simulink model "complex_addsub_test"  (Simulink 7.0)
settings: Solver=VariableStepDiscrete  StartTime=0.0  StopTime=1000  RelTol=1e-3
libraries: xbsIndex_r4 x13, casper_library x5
settings Model: Creator=User  LastModifiedBy=User
settings DebuggingCC: SaveWithDisabledLinksMsg=none  SaveWithParameterizedLinksMsg=none

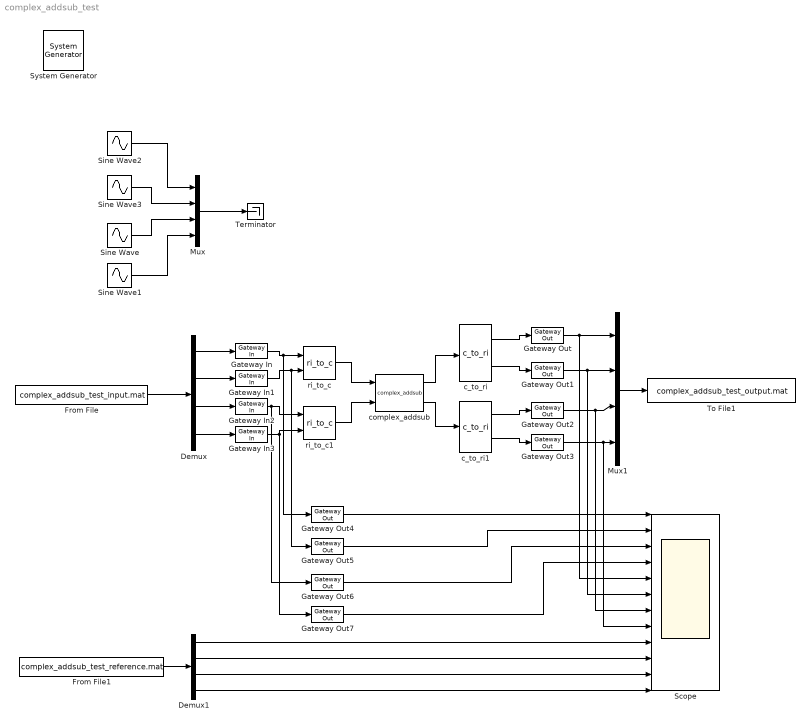
== system complex_addsub_test ==
  " System Generator" : xbsIndex_r4/ System Generator  Tag=genX  SystemSampleTime=-1  xilinxfamily=Virtex4  part=xc4vsx35  speed=-10  package=ff668  synthesis_tool=XST  clock_wrapper=Clock Enables  directory=./netlist  testbench=off  simulink_period=1  sysclk_period=100  dcm_input_clock_period=100  incr_netlist=off  trim_vbits=Everywhere in SubSystem  dbl_ovrd=According to Block Masks  core_generation=According to Block Masks  run_coregen=off  deprecated_control=off  eval_field=0  block_type=sysgen
      settings: block_version=10.1.1
  Demux : Demux
  Demux1 : Demux
  From File : FromFile  FileName=complex_addsub_test_input.mat  SampleTime=1
  From File1 : FromFile  FileName=complex_addsub_test_reference.mat  SampleTime=1
  Gateway In{,1..3} (4 alike) : xbsIndex_r4/Gateway In  arith_type="Signed  (2's comp)"  n_bits=12  bin_pt=11  quantization=Truncate  overflow=Wrap  period=1  dbl_ovrd=off  timing_constraint=None  locs_specified=off  LOCs={}  block_type=gatewayin
      settings: infoedit="Gateway in block.  Converts inputs of type Simulink integer, double and fixed point to  Xilinx fixed point type.<P><P>Hardware notes:  In hardware these blocks become top level input ports."  block_version=10.1.1
  Gateway Out{,1..7} (8 alike) : xbsIndex_r4/Gateway Out  hdl_port=on  timing_constraint=None  locs_specified=off  LOCs={}  block_type=gatewayout
      settings: infoedit="Gateway out block.  Converts Xilinx fixed point inputs into ouputs of type Simulink integer, double, or fixed point.<P><P>Hardware notes:  In hardware these blocks become top level output ports or are discarded, depending on how they are configured."  block_version=10.1.1
  Mux : Mux
  Mux1 : Mux
  Scope : Scope  NumInputPorts=12
      settings: YMin=-5~-5~-5~-5~-5~-5~-5~-5~-5~-5~-5~-5  YMax=5~5~5~5~5~5~5~5~5~5~5~5
  Sine Wave : Sin  SineType=Sample based  Samples=123  SampleTime=1
  Sine Wave1 : Sin  SineType=Sample based  Samples=67  SampleTime=1
  Sine Wave2 : Sin  SineType=Sample based  Samples=111  SampleTime=1
  Sine Wave3 : Sin  SineType=Sample based  Samples=99  SampleTime=1
  Terminator : Terminator
  To File1 : ToFile  Filename=complex_addsub_test_output.mat  MatrixName=output
  c_to_ri : casper_library/Misc/c_to_ri  SystemSampleTime=-1  n_bits=12  bin_pt=11
      settings: AttributesFormatString=12_11 r/i
  c_to_ri1 : casper_library/Misc/c_to_ri  SystemSampleTime=-1  n_bits=12  bin_pt=11
      settings: AttributesFormatString=12_11 r/i
  complex_addsub : casper_library/Misc/complex_addsub  SystemSampleTime=-1  BitWidth=12  add_latency=3
  ri_to_c : casper_library/Misc/ri_to_c  SystemSampleTime=-1
  ri_to_c1 : casper_library/Misc/ri_to_c  SystemSampleTime=-1
  wires:
  Sine Wave2/1 -> Mux/1
  Sine Wave3/1 -> Mux/2
  Sine Wave/1 -> Mux/3
  Sine Wave1/1 -> Mux/4
  Mux/1 -> Terminator/1
  From File/1 -> Demux/1
  Demux/1 -> Gateway In/1
  Demux/2 -> Gateway In1/1
  Demux/3 -> Gateway In2/1
  Demux/4 -> Gateway In3/1
  Gateway In/1 -> ri_to_c/1, Gateway Out4/1
  Gateway In1/1 -> ri_to_c/2, Gateway Out5/1
  Gateway In2/1 -> ri_to_c1/1, Gateway Out6/1
  Gateway In3/1 -> ri_to_c1/2, Gateway Out7/1
  ri_to_c/1 -> complex_addsub/1
  ri_to_c1/1 -> complex_addsub/2
  complex_addsub/1 -> c_to_ri/1
  complex_addsub/2 -> c_to_ri1/1
  c_to_ri/1 -> Gateway Out/1
  c_to_ri/2 -> Gateway Out1/1
  c_to_ri1/1 -> Gateway Out2/1
  c_to_ri1/2 -> Gateway Out3/1
  Gateway Out/1 -> Mux1/1, Scope/5
  Gateway Out1/1 -> Mux1/2, Scope/6
  Gateway Out2/1 -> Mux1/3, Scope/7
  Gateway Out3/1 -> Mux1/4, Scope/8
  Mux1/1 -> To File1/1
  From File1/1 -> Demux1/1
  Gateway Out4/1 -> Scope/1
  Gateway Out5/1 -> Scope/2
  Gateway Out6/1 -> Scope/3
  Gateway Out7/1 -> Scope/4
  Demux1/1 -> Scope/9
  Demux1/2 -> Scope/10
  Demux1/3 -> Scope/11
  Demux1/4 -> Scope/12
